simulink model "Copy_of_GS_Aircraft"  (R2022b)
settings: Solver=VariableStepAuto  StartTime=0.0  StopTime=140  RelTol=1e-3
values from neighbouring files (symbols this model uses):
  gs_ref_angle = gs_angle_deg/180*pi    (= 0.0523598775598)    [FindF16Dynamics.m]
  h_flare = 19.2    [FindF16Dynamics.m]
  SS_long_lo_GS_red = ss(A_long_ac_GS, B_long_ac_GS, SS_lo.C(GS_outputs,GS_states(1:5)), SS_lo.D(GS_outputs,GS_inputs))    [FindF16Dynamics.m]
  start_pos = 2000/tan(gs_ref_angle) + 10*velocity    [FindF16Dynamics.m]
  tau = 1.22    [FindF16Dynamics.m]    (also in parameters_calc.m = 35.9712230216)
undefined symbols (not defined in the file or in its folder): trim_control_lo, trim_thrust_lo
libraries: slpidlib x4, simulink_extras x2
settings Model: Creator=alec-  LastModifiedBy=alec-

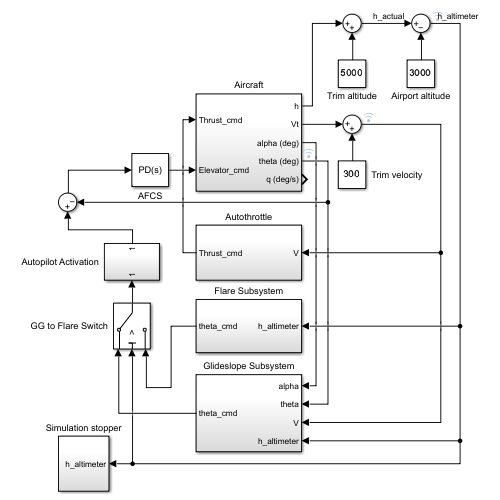
[thumbnail: Simulink's stored preview of the top-level diagram]
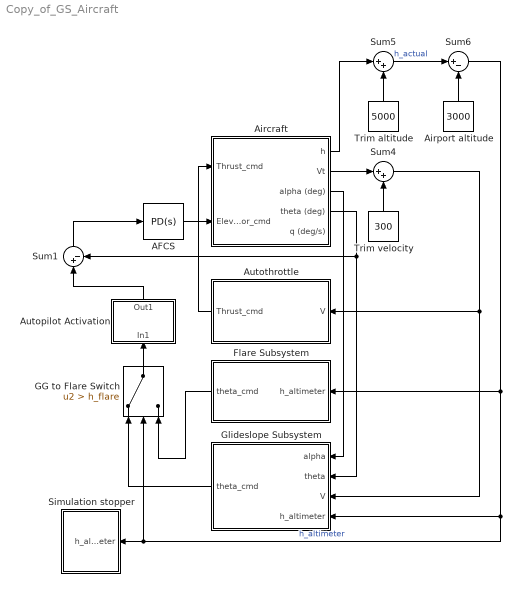
== system Copy_of_GS_Aircraft ==
  AFCS : slpidlib/PID Controller  Controller=PD  Form=Parallel  TimeDomain=Continuous-time  UseExternalTs=off  SampleTime=-1  IntegratorMethod=Forward Euler  FilterMethod=Forward Euler  ControllerParametersSource=internal  P=-25  I=0  UseKiTs=off  D=-7  N=100  UseFilter=on  TunerSelectOption=Transfer Function Based (PID Tuner App)  InitialConditionSource=internal  InitialConditionForIntegrator=0  InitialConditionForFilter=0  DifferentiatorICPrevScaledInput=0  ExternalReset=none  TrackingMode=off  Kt=1  LimitOutput=off  SatLimitsSource=internal  UpperSaturationLimit=inf  LowerSaturationLimit=-inf  LinearizeAsGain=on  AntiWindupMode=none  Kb=1  LimitIntegrator=off  UpperIntegratorSaturationLimit=inf  LowerIntegratorSaturationLimit=-inf  POutMin=[]  POutMax=[]  IOutMin=[]  IOutMax=[]  DOutMin=[]  DOutMax=[]  NOutMin=[]  NOutMax=[]  SumOutMin=[]  SumOutMax=[]  SaturationOutMin=[]  SaturationOutMax=[]  PParamMin=[]  PParamMax=[]  IParamMin=[]  IParamMax=[]  DParamMin=[]  DParamMax=[]  NParamMin=[]  NParamMax=[]  KbParamMin=[]  KbParamMax=[]  KtParamMin=[]  KtParamMax=[]  KbOutMin=[]  KbOutMax=[]  KtOutMin=[]  KtOutMax=[]  IntegratorOutMin=[]  IntegratorOutMax=[]  FilterOutMin=[]  FilterOutMax=[]  SumI1OutMin=[]  SumI1OutMax=[]  SumI2OutMin=[]  SumI2OutMax=[]  SumI3OutMin=[]  SumI3OutMax=[]  SumI4OutMin=[]  SumI4OutMax=[]  SumDOutMin=[]  SumDOutMax=[]  DifferentiatorOutMin=[]  DifferentiatorOutMax=[]  FilterDiffOutCoefMin=[]  FilterDiffOutCoefMax=[]  ReciprocalOutMin=[]  ReciprocalOutMax=[]  SumDenOutMin=[]  SumDenOutMax=[]  SumNumOutMin=[]  SumNumOutMax=[]  DivideOutMin=[]  DivideOutMax=[]  UdiffTsProdOutMin=[]  UdiffTsProdOutMax=[]  NTsProdOutMin=[]  NTsProdOutMax=[]  UintegralTsProdOutMin=[]  UintegralTsProdOutMax=[]  UngainTsProdOutMin=[]  UngainTsProdOutMax=[]  ClampingZeroOutDataTypeStr=Inherit: Inherit via back propagation  ClampingZeroOutMin=[]  ClampingZeroOutMax=[]  FilterDenConstantOutDataTypeStr=Inherit: Inherit via back propagation  FilterDenConstantOutMin=[]  FilterDenConstantOutMax=[]  PCopyOutDataTypeStr=Inherit: Inherit via back propagation  PCopyOutMin=[]  PCopyOutMax=[]  NCopyOutDataTypeStr=Inherit: Inherit via back propagation  NCopyOutMin=[]  NCopyOutMax=[]  IntegratorContinuousStateAttributes=''  IntegratorStateMustResolveToSignalObject=off  IntegratorRTWStateStorageClass=Auto  FilterContinuousStateAttributes=''  FilterStateMustResolveToSignalObject=off  FilterRTWStateStorageClass=Auto  ParallelPVariant=InternalParameters  IdealPVariant=Disabled  IVariant=Disabled  DVariant=InternalParameters  IntegratorVariant=Disabled  SatVariant=Disabled  AWVariant=Disabled  PCopyVariant=Disabled  TRVariant=Disabled  FdbkBlocksVariant=Forward  IdealPFdbkVariant=Disabled  SatFdbkVariant=Disabled  DerivativeFilterVariant=ContFilter  NVariant=InternalParameters  NCopyVariant=Disabled  FilterICVariant=InternalICsFilter  IntegratorICVariant=Disabled  ExternalResetVariant=Disabled  TRSumVariant=Passthrough  SumFdbkVariant=Disabled  SumVariant=Sum_PD  TsampFilterVariant=InternalTs  TsampNgainVariant=Passthrough  TsampIntegralVariant=Disabled_SignalSpec  ExternalSaturationOutDataTypeStr=Inherit: Same as second input
  Aircraft : Subsystem
  Airport altitude : Constant  Value=3000
  Autopilot Activation : Subsystem
  Autothrottle : Subsystem
  Flare Subsystem : Subsystem
  GG to Flare Switch : Switch  Criteria=u2 > Threshold  Threshold=h_flare  SaturateOnIntegerOverflow=off  InputSameDT=off
  Glideslope Subsystem : Subsystem
  Simulation stopper : Subsystem
  Sum1 : Sum  Inputs=|+-
  Sum4 : Sum  Inputs=|++
  Sum5 : Sum  Inputs=|++
  Sum6 : Sum  Inputs=|+-
  Trim altitude : Constant  Value=5000
  Trim velocity : Constant  Value=300
  wires:
  Aircraft/4(theta (deg)) -> Glideslope Subsystem/2(theta), Sum1/2
  Sum1/1 -> AFCS/1
  Trim velocity/1 -> Sum4/2
  Aircraft/2(Vt) -> Sum4/1
  Sum4/1 -> Glideslope Subsystem/3(V), Autothrottle/1(V)
  Aircraft/1(h) -> Sum5/1
  Trim altitude/1 -> Sum5/2
  Sum5/1 -> Sum6/1  "h_actual"
  Airport altitude/1 -> Sum6/2
  Sum6/1 -> GG to Flare Switch/2, Simulation stopper/1(h_altimeter), Glideslope Subsystem/4(h_altimeter), Flare Subsystem/1(h_altimeter)  "h_altimeter"
  Glideslope Subsystem/1(theta_cmd) -> GG to Flare Switch/1
  AFCS/1 -> Aircraft/2(Elevator_cmd)
  Autothrottle/1(Thrust_cmd) -> Aircraft/1(Thrust_cmd)
  Aircraft/3(alpha (deg)) -> Glideslope Subsystem/1(alpha)
  GG to Flare Switch/1 -> Autopilot Activation/1(In1)
  Autopilot Activation/1(Out1) -> Sum1/1
  Flare Subsystem/1(theta_cmd) -> GG to Flare Switch/3

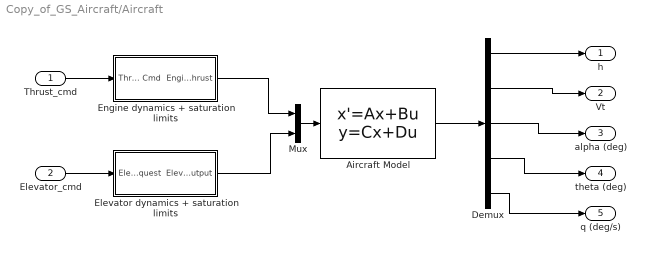
== system Copy_of_GS_Aircraft/Aircraft ==
  Thrust_cmd : Inport
  Elevator_cmd : Inport  Port=2
  Aircraft Model : StateSpace  A=SS_long_lo_GS_red.A  B=SS_long_lo_GS_red.B  C=SS_long_lo_GS_red.C  D=SS_long_lo_GS_red.D  InitialCondition=0
  Demux : Demux  Outputs=5
  Elevator dynamics + saturation limits : Subsystem
  Engine dynamics + saturation limits : Subsystem
  Mux : Mux  Inputs=2
  h : Outport
  Vt : Outport  Port=2
  alpha (deg) : Outport  Port=3
  theta (deg) : Outport  Port=4
  q (deg/s) : Outport  Port=5
  wires:
  Demux/2 -> Vt/1
  Demux/1 -> h/1
  Elevator dynamics + saturation limits/1(Elevator actuator output) -> Mux/2
  Mux/1 -> Aircraft Model/1
  Engine dynamics + saturation limits/1(Engine Thrust) -> Mux/1
  Aircraft Model/1 -> Demux/1
  Thrust_cmd/1 -> Engine dynamics + saturation limits/1(Thrust Cmd)
  Demux/3 -> alpha (deg)/1
  Elevator_cmd/1 -> Elevator dynamics + saturation limits/1(Elevator_cmd request)
  Demux/4 -> theta (deg)/1
  Demux/5 -> q (deg/s)/1

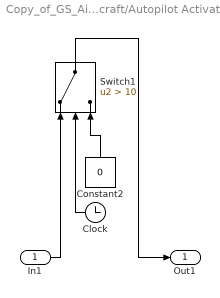
== system Copy_of_GS_Aircraft/Autopilot Activation ==
  In1 : Inport
  Clock : Clock
  Constant2 : Constant  Value=0
  Switch1 : Switch  Criteria=u2 > Threshold  Threshold=10  SaturateOnIntegerOverflow=off  InputSameDT=off
  Out1 : Outport
  wires:
  Constant2/1 -> Switch1/3
  Clock/1 -> Switch1/2
  Switch1/1 -> Out1/1
  In1/1 -> Switch1/1

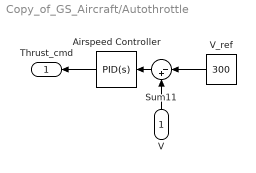
== system Copy_of_GS_Aircraft/Autothrottle ==
  V : Inport
  Airspeed Controller : slpidlib/PID Controller  Controller=PID  Form=Parallel  TimeDomain=Continuous-time  UseExternalTs=off  SampleTime=-1  IntegratorMethod=Forward Euler  FilterMethod=Forward Euler  ControllerParametersSource=internal  P=-1000  I=-200  UseKiTs=off  D=-200  N=100  UseFilter=on  TunerSelectOption=Transfer Function Based (PID Tuner App)  InitialConditionSource=internal  InitialConditionForIntegrator=0  InitialConditionForFilter=0  DifferentiatorICPrevScaledInput=0  ExternalReset=none  TrackingMode=off  Kt=1  LimitOutput=off  SatLimitsSource=internal  UpperSaturationLimit=inf  LowerSaturationLimit=-inf  LinearizeAsGain=on  AntiWindupMode=none  Kb=1  LimitIntegrator=off  UpperIntegratorSaturationLimit=inf  LowerIntegratorSaturationLimit=-inf  POutMin=[]  POutMax=[]  IOutMin=[]  IOutMax=[]  DOutMin=[]  DOutMax=[]  NOutMin=[]  NOutMax=[]  SumOutMin=[]  SumOutMax=[]  SaturationOutMin=[]  SaturationOutMax=[]  PParamMin=[]  PParamMax=[]  IParamMin=[]  IParamMax=[]  DParamMin=[]  DParamMax=[]  NParamMin=[]  NParamMax=[]  KbParamMin=[]  KbParamMax=[]  KtParamMin=[]  KtParamMax=[]  KbOutMin=[]  KbOutMax=[]  KtOutMin=[]  KtOutMax=[]  IntegratorOutMin=[]  IntegratorOutMax=[]  FilterOutMin=[]  FilterOutMax=[]  SumI1OutMin=[]  SumI1OutMax=[]  SumI2OutMin=[]  SumI2OutMax=[]  SumI3OutMin=[]  SumI3OutMax=[]  SumI4OutMin=[]  SumI4OutMax=[]  SumDOutMin=[]  SumDOutMax=[]  DifferentiatorOutMin=[]  DifferentiatorOutMax=[]  FilterDiffOutCoefMin=[]  FilterDiffOutCoefMax=[]  ReciprocalOutMin=[]  ReciprocalOutMax=[]  SumDenOutMin=[]  SumDenOutMax=[]  SumNumOutMin=[]  SumNumOutMax=[]  DivideOutMin=[]  DivideOutMax=[]  UdiffTsProdOutMin=[]  UdiffTsProdOutMax=[]  NTsProdOutMin=[]  NTsProdOutMax=[]  UintegralTsProdOutMin=[]  UintegralTsProdOutMax=[]  UngainTsProdOutMin=[]  UngainTsProdOutMax=[]  ClampingZeroOutDataTypeStr=Inherit: Inherit via back propagation  ClampingZeroOutMin=[]  ClampingZeroOutMax=[]  FilterDenConstantOutDataTypeStr=Inherit: Inherit via back propagation  FilterDenConstantOutMin=[]  FilterDenConstantOutMax=[]  PCopyOutDataTypeStr=Inherit: Inherit via back propagation  PCopyOutMin=[]  PCopyOutMax=[]  NCopyOutDataTypeStr=Inherit: Inherit via back propagation  NCopyOutMin=[]  NCopyOutMax=[]  IntegratorContinuousStateAttributes=''  IntegratorStateMustResolveToSignalObject=off  IntegratorRTWStateStorageClass=Auto  FilterContinuousStateAttributes=''  FilterStateMustResolveToSignalObject=off  FilterRTWStateStorageClass=Auto  ParallelPVariant=InternalParameters  IdealPVariant=Disabled  IVariant=InternalParameters  DVariant=InternalParameters  IntegratorVariant=Continuous  SatVariant=Disabled  AWVariant=Passthrough  PCopyVariant=Disabled  TRVariant=Disabled  FdbkBlocksVariant=Forward  IdealPFdbkVariant=Disabled  SatFdbkVariant=Disabled  DerivativeFilterVariant=ContFilter  NVariant=InternalParameters  NCopyVariant=Disabled  FilterICVariant=InternalICsFilter  IntegratorICVariant=InternalICs  ExternalResetVariant=Disabled  TRSumVariant=Passthrough  SumFdbkVariant=Disabled  SumVariant=Sum_PID  TsampFilterVariant=InternalTs  TsampNgainVariant=Passthrough  TsampIntegralVariant=Passthrough  ExternalSaturationOutDataTypeStr=Inherit: Same as second input
  Sum11 : Sum  Inputs=|-+
  V_ref : Constant  Value=300
  Thrust_cmd : Outport
  wires:
  V/1 -> Sum11/2
  V_ref/1 -> Sum11/1
  Sum11/1 -> Airspeed Controller/1
  Airspeed Controller/1 -> Thrust_cmd/1

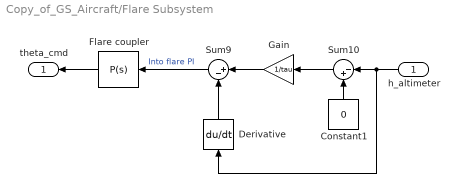
== system Copy_of_GS_Aircraft/Flare Subsystem ==
  h_altimeter : Inport
  Constant1 : Constant  Value=0
  Derivative : Derivative
  Flare coupler : slpidlib/PID Controller  Controller=P  Form=Parallel  TimeDomain=Continuous-time  UseExternalTs=off  SampleTime=-1  IntegratorMethod=Forward Euler  FilterMethod=Forward Euler  ControllerParametersSource=internal  P=0.08  I=0  UseKiTs=off  D=0  N=100  UseFilter=on  TunerSelectOption=Transfer Function Based (PID Tuner App)  InitialConditionSource=internal  InitialConditionForIntegrator=0  InitialConditionForFilter=0  DifferentiatorICPrevScaledInput=0  ExternalReset=none  TrackingMode=off  Kt=1  LimitOutput=off  SatLimitsSource=internal  UpperSaturationLimit=inf  LowerSaturationLimit=-inf  LinearizeAsGain=on  AntiWindupMode=none  Kb=1  LimitIntegrator=off  UpperIntegratorSaturationLimit=inf  LowerIntegratorSaturationLimit=-inf  POutMin=[]  POutMax=[]  IOutMin=[]  IOutMax=[]  DOutMin=[]  DOutMax=[]  NOutMin=[]  NOutMax=[]  SumOutMin=[]  SumOutMax=[]  SaturationOutMin=[]  SaturationOutMax=[]  PParamMin=[]  PParamMax=[]  IParamMin=[]  IParamMax=[]  DParamMin=[]  DParamMax=[]  NParamMin=[]  NParamMax=[]  KbParamMin=[]  KbParamMax=[]  KtParamMin=[]  KtParamMax=[]  KbOutMin=[]  KbOutMax=[]  KtOutMin=[]  KtOutMax=[]  IntegratorOutMin=[]  IntegratorOutMax=[]  FilterOutMin=[]  FilterOutMax=[]  SumI1OutMin=[]  SumI1OutMax=[]  SumI2OutMin=[]  SumI2OutMax=[]  SumI3OutMin=[]  SumI3OutMax=[]  SumI4OutMin=[]  SumI4OutMax=[]  SumDOutMin=[]  SumDOutMax=[]  DifferentiatorOutMin=[]  DifferentiatorOutMax=[]  FilterDiffOutCoefMin=[]  FilterDiffOutCoefMax=[]  ReciprocalOutMin=[]  ReciprocalOutMax=[]  SumDenOutMin=[]  SumDenOutMax=[]  SumNumOutMin=[]  SumNumOutMax=[]  DivideOutMin=[]  DivideOutMax=[]  UdiffTsProdOutMin=[]  UdiffTsProdOutMax=[]  NTsProdOutMin=[]  NTsProdOutMax=[]  UintegralTsProdOutMin=[]  UintegralTsProdOutMax=[]  UngainTsProdOutMin=[]  UngainTsProdOutMax=[]  ClampingZeroOutDataTypeStr=Inherit: Inherit via back propagation  ClampingZeroOutMin=[]  ClampingZeroOutMax=[]  FilterDenConstantOutDataTypeStr=Inherit: Inherit via back propagation  FilterDenConstantOutMin=[]  FilterDenConstantOutMax=[]  PCopyOutDataTypeStr=Inherit: Inherit via back propagation  PCopyOutMin=[]  PCopyOutMax=[]  NCopyOutDataTypeStr=Inherit: Inherit via back propagation  NCopyOutMin=[]  NCopyOutMax=[]  IntegratorContinuousStateAttributes=''  IntegratorStateMustResolveToSignalObject=off  IntegratorRTWStateStorageClass=Auto  FilterContinuousStateAttributes=''  FilterStateMustResolveToSignalObject=off  FilterRTWStateStorageClass=Auto  ParallelPVariant=InternalParameters  IdealPVariant=Disabled  IVariant=Disabled  DVariant=Disabled  IntegratorVariant=Disabled  SatVariant=Disabled  AWVariant=Disabled  PCopyVariant=Disabled  TRVariant=Disabled  FdbkBlocksVariant=Forward  IdealPFdbkVariant=Disabled  SatFdbkVariant=Disabled  DerivativeFilterVariant=Disabled  NVariant=Disabled  NCopyVariant=Disabled_SignalSpec  FilterICVariant=Disabled  IntegratorICVariant=Disabled  ExternalResetVariant=Disabled  TRSumVariant=Passthrough  SumFdbkVariant=Disabled  SumVariant=Passthrough_P  TsampFilterVariant=InternalTs  TsampNgainVariant=Passthrough  TsampIntegralVariant=Disabled_SignalSpec  ExternalSaturationOutDataTypeStr=Inherit: Same as second input
  Gain : Gain  Gain=1/tau
  Sum10 : Sum  Inputs=|-+
  Sum9 : Sum  Inputs=|+-
  theta_cmd : Outport
  wires:
  Sum10/1 -> Gain/1
  Gain/1 -> Sum9/1
  Constant1/1 -> Sum10/2
  h_altimeter/1 -> Derivative/1, Sum10/1
  Flare coupler/1 -> theta_cmd/1
  Derivative/1 -> Sum9/2
  Sum9/1 -> Flare coupler/1  "Into flare PI"

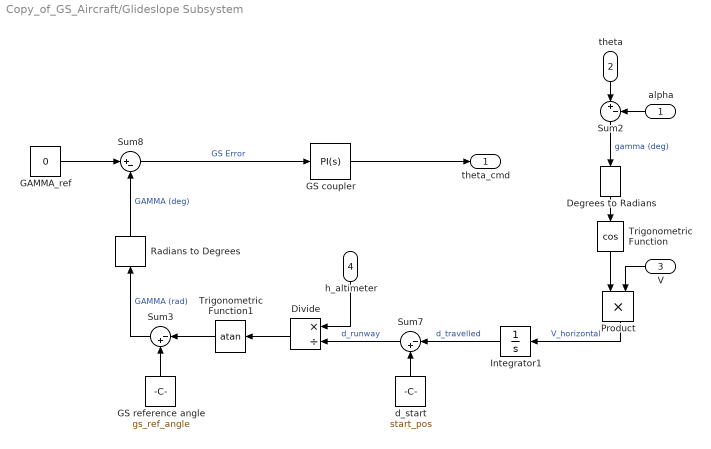
== system Copy_of_GS_Aircraft/Glideslope Subsystem ==
  alpha : Inport
  theta : Inport  Port=2
  V : Inport  Port=3
  h_altimeter : Inport  Port=4
  Degrees to Radians : simulink_extras/Transformations/Degrees to Radians
  Divide : Product  Inputs=*/
  GAMMA_ref : Constant  Value=0
  GS coupler : slpidlib/PID Controller  Controller=PI  Form=Parallel  TimeDomain=Continuous-time  UseExternalTs=off  SampleTime=-1  IntegratorMethod=Forward Euler  FilterMethod=Forward Euler  ControllerParametersSource=internal  P=-80  I=-5  UseKiTs=off  D=0  N=100  UseFilter=on  TunerSelectOption=Transfer Function Based (PID Tuner App)  InitialConditionSource=internal  InitialConditionForIntegrator=0  InitialConditionForFilter=0  DifferentiatorICPrevScaledInput=0  ExternalReset=none  TrackingMode=off  Kt=1  LimitOutput=off  SatLimitsSource=internal  UpperSaturationLimit=inf  LowerSaturationLimit=-inf  LinearizeAsGain=on  AntiWindupMode=none  Kb=1  LimitIntegrator=off  UpperIntegratorSaturationLimit=inf  LowerIntegratorSaturationLimit=-inf  POutMin=[]  POutMax=[]  IOutMin=[]  IOutMax=[]  DOutMin=[]  DOutMax=[]  NOutMin=[]  NOutMax=[]  SumOutMin=[]  SumOutMax=[]  SaturationOutMin=[]  SaturationOutMax=[]  PParamMin=[]  PParamMax=[]  IParamMin=[]  IParamMax=[]  DParamMin=[]  DParamMax=[]  NParamMin=[]  NParamMax=[]  KbParamMin=[]  KbParamMax=[]  KtParamMin=[]  KtParamMax=[]  KbOutMin=[]  KbOutMax=[]  KtOutMin=[]  KtOutMax=[]  IntegratorOutMin=[]  IntegratorOutMax=[]  FilterOutMin=[]  FilterOutMax=[]  SumI1OutMin=[]  SumI1OutMax=[]  SumI2OutMin=[]  SumI2OutMax=[]  SumI3OutMin=[]  SumI3OutMax=[]  SumI4OutMin=[]  SumI4OutMax=[]  SumDOutMin=[]  SumDOutMax=[]  DifferentiatorOutMin=[]  DifferentiatorOutMax=[]  FilterDiffOutCoefMin=[]  FilterDiffOutCoefMax=[]  ReciprocalOutMin=[]  ReciprocalOutMax=[]  SumDenOutMin=[]  SumDenOutMax=[]  SumNumOutMin=[]  SumNumOutMax=[]  DivideOutMin=[]  DivideOutMax=[]  UdiffTsProdOutMin=[]  UdiffTsProdOutMax=[]  NTsProdOutMin=[]  NTsProdOutMax=[]  UintegralTsProdOutMin=[]  UintegralTsProdOutMax=[]  UngainTsProdOutMin=[]  UngainTsProdOutMax=[]  ClampingZeroOutDataTypeStr=Inherit: Inherit via back propagation  ClampingZeroOutMin=[]  ClampingZeroOutMax=[]  FilterDenConstantOutDataTypeStr=Inherit: Inherit via back propagation  FilterDenConstantOutMin=[]  FilterDenConstantOutMax=[]  PCopyOutDataTypeStr=Inherit: Inherit via back propagation  PCopyOutMin=[]  PCopyOutMax=[]  NCopyOutDataTypeStr=Inherit: Inherit via back propagation  NCopyOutMin=[]  NCopyOutMax=[]  IntegratorContinuousStateAttributes=''  IntegratorStateMustResolveToSignalObject=off  IntegratorRTWStateStorageClass=Auto  FilterContinuousStateAttributes=''  FilterStateMustResolveToSignalObject=off  FilterRTWStateStorageClass=Auto  ParallelPVariant=InternalParameters  IdealPVariant=Disabled  IVariant=InternalParameters  DVariant=Disabled  IntegratorVariant=Continuous  SatVariant=Disabled  AWVariant=Passthrough  PCopyVariant=Disabled  TRVariant=Disabled  FdbkBlocksVariant=Forward  IdealPFdbkVariant=Disabled  SatFdbkVariant=Disabled  DerivativeFilterVariant=Disabled  NVariant=Disabled  NCopyVariant=Disabled_SignalSpec  FilterICVariant=Disabled  IntegratorICVariant=InternalICs  ExternalResetVariant=Disabled  TRSumVariant=Passthrough  SumFdbkVariant=Disabled  SumVariant=Sum_PI  TsampFilterVariant=InternalTs  TsampNgainVariant=Passthrough  TsampIntegralVariant=Passthrough  ExternalSaturationOutDataTypeStr=Inherit: Same as second input
  GS reference angle : Constant  Value=gs_ref_angle
  Integrator1 : Integrator
  Product : Product
  Radians to Degrees : simulink_extras/Transformations/Radians to Degrees
  Sum2 : Sum  Inputs=|+-
  Sum3 : Sum  Inputs=|-+
  Sum7 : Sum  Inputs=|-+
  Sum8 : Sum  Inputs=|+-
  Trigonometric Function : Trigonometry  Operator=cos
  Trigonometric Function1 : Trigonometry  Operator=atan
  d_start : Constant  Value=start_pos
  theta_cmd : Outport
  wires:
  d_start/1 -> Sum7/2
  V/1 -> Product/2
  GS reference angle/1 -> Sum3/2
  Degrees to Radians/1 -> Trigonometric Function/1
  Product/1 -> Integrator1/1  "V_horizontal"
  Sum7/1 -> Divide/2  "d_runway"
  GAMMA_ref/1 -> Sum8/1
  Trigonometric Function/1 -> Product/1
  Divide/1 -> Trigonometric Function1/1
  Sum3/1 -> Radians to Degrees/1  "GAMMA (rad)"
  Sum2/1 -> Degrees to Radians/1  "gamma (deg)"
  Integrator1/1 -> Sum7/1  "d_travelled"
  Radians to Degrees/1 -> Sum8/2  "GAMMA (deg)"
  Trigonometric Function1/1 -> Sum3/1
  h_altimeter/1 -> Divide/1
  theta/1 -> Sum2/1
  alpha/1 -> Sum2/2
  GS coupler/1 -> theta_cmd/1
  Sum8/1 -> GS coupler/1  "GS Error"

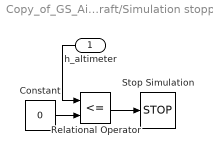
== system Copy_of_GS_Aircraft/Simulation stopper ==
  h_altimeter : Inport
  Constant : Constant  Value=0
  Relational Operator : RelationalOperator  Operator=<=  OutDataTypeStr=boolean  RndMeth=Simplest  InputSameDT=off
  Stop Simulation : Stop
  wires:
  Constant/1 -> Relational Operator/2
  Relational Operator/1 -> Stop Simulation/1
  h_altimeter/1 -> Relational Operator/1

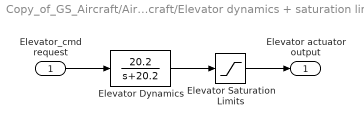
== system Copy_of_GS_Aircraft/Aircraft/Elevator dynamics + saturation limits ==
  Elevator_cmd request : Inport
  Elevator Dynamics : TransferFcn  Numerator=[20.2]  Denominator=[1 20.2]
  Elevator Saturation Limits : Saturate  UpperLimit=25-trim_control_lo(1)  LowerLimit=-25-trim_control_lo(1)
  Elevator actuator output : Outport
  wires:
  Elevator_cmd request/1 -> Elevator Dynamics/1
  Elevator Dynamics/1 -> Elevator Saturation Limits/1
  Elevator Saturation Limits/1 -> Elevator actuator output/1

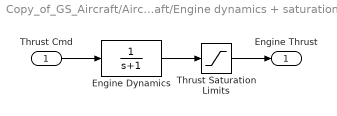
== system Copy_of_GS_Aircraft/Aircraft/Engine dynamics + saturation limits ==
  Thrust Cmd : Inport
  Engine Dynamics : TransferFcn  Denominator=[1 1]
  Thrust Saturation Limits : Saturate  UpperLimit=19000-trim_thrust_lo  LowerLimit=1000-trim_thrust_lo
  Engine Thrust : Outport
  wires:
  Thrust Cmd/1 -> Engine Dynamics/1
  Engine Dynamics/1 -> Thrust Saturation Limits/1
  Thrust Saturation Limits/1 -> Engine Thrust/1
